simulink model "modelo_fibonacci"  (R2023b)
settings: Solver=FixedStepDiscrete  StartTime=1  StopTime=8  FixedStep=1  RelTol=1e-3
settings Model: Creator=alfre  LastModifiedBy=alfre

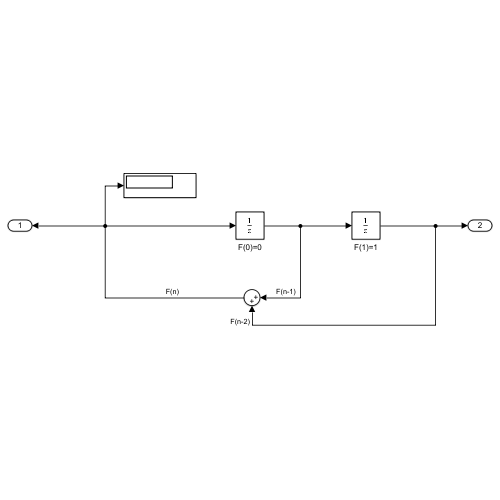
[thumbnail: Simulink's stored preview of the top-level diagram]
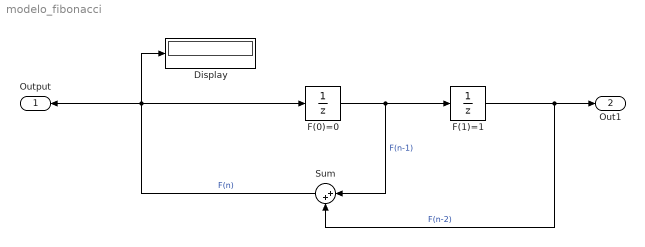
== system modelo_fibonacci ==
  Display : Display
      settings: Format=decimal (Stored Integer)
  F(0)=0 : UnitDelay  SampleTime=-1  HasFrameUpgradeWarning=on
  F(1)=1 : UnitDelay  InitialCondition=1  SampleTime=-1  HasFrameUpgradeWarning=on
  Sum : Sum  Inputs=|++
  Output : Outport
  Out1 : Outport  Port=2
  wires:
  Sum/1 -> Output/1, F(0)=0/1, Display/1  "F(n)"
  F(0)=0/1 -> Sum/1, F(1)=1/1  "F(n-1)"
  F(1)=1/1 -> Out1/1, Sum/2  "F(n-2)"
